simulink model "sfcndemo_dtype_io"  (Simulink 6.0)
settings: Solver=FixedStepDiscrete  StartTime=0.0  StopTime=10.0  RelTol=1e-3
settings Model: Creator=The MathWorks Inc.  LastModifiedBy=batserve  ExtModeAutoUpdateStatusClock=off
settings OptimizationCC: BlockReduction=off  BooleanDataType=off
settings DebuggingCC: CheckExecutionContextPreStartOutputMsg=on  CheckExecutionContextRuntimeOutputMsg=on  SolverPrmCheckMsg=none
settings HardwareCC: TargetUnknown=on

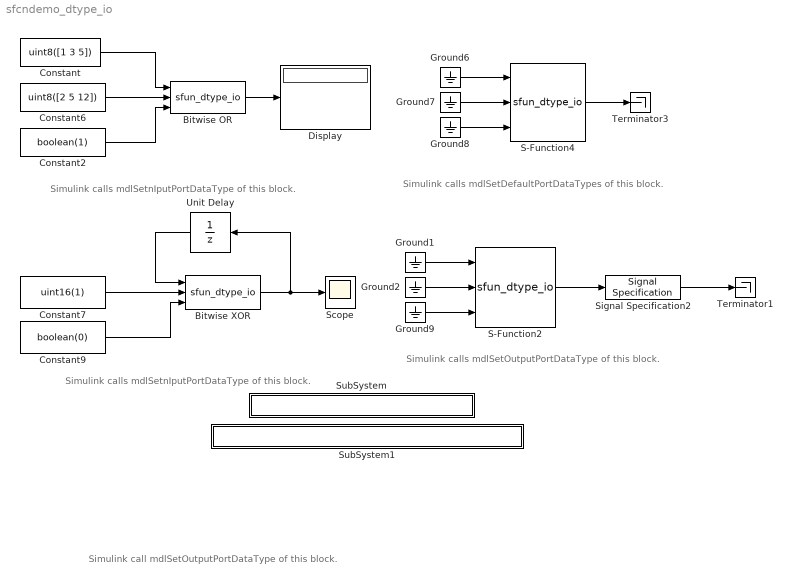
== system sfcndemo_dtype_io ==
  note: Simulink calls mdlSetDefaultPortDataTypes of this block.
  note: Simulink calls mdlSetOutputPortDataType of this block.
  note: Simulink call mdlSetOutputPortDataType of this block.
  note: Simulink calls mdlSetnIputPortDataType of this block.
  note: Simulink calls mdlSetnIputPortDataType of this block.
  Bitwise OR : S-Function  FunctionName=sfun_dtype_io
  Bitwise XOR : S-Function  FunctionName=sfun_dtype_io
  Constant : Constant  Value=uint8([1 3 5])
  Constant2 : Constant  Value=boolean(1)
  Constant6 : Constant  Value=uint8([2 5 12])
  Constant7 : Constant  Value=uint16(1)
  Constant9 : Constant  Value=boolean(0)
  Display : Display
  Ground{1..2,6..9} (6 alike) : Ground
  S-Function2 : S-Function  FunctionName=sfun_dtype_io
  S-Function4 : S-Function  FunctionName=sfun_dtype_io
  Scope : Scope
  Signal Specification2 : SignalSpecification  DataType=uint32
  SubSystem : Subsystem  PropExecContextAcrossSSBoundary=on
      settings: OpenFcn=edit(fullfile(matlabroot,'simulink','src','sfun_dtype_io.c'))
      mask Display: disp('matlabroot\simulink\src\sfun_dtype_io.c');
  SubSystem1 : Subsystem  PropExecContextAcrossSSBoundary=on
      settings: OpenFcn=edit(fullfile(matlabroot,'toolbox','simulink','blocks','tlc_c','sfun_dtype_io.tlc'))
      mask Display: disp('matlabroot\toolbox\simulink\blocks\tlc_c\sfun_dtype_io.tlc');
  Terminator1 : Terminator
  Terminator3 : Terminator
  Unit Delay : UnitDelay  Orientation=left
  wires:
  Constant/1 -> Bitwise OR/1
  Bitwise OR/1 -> Display/1
  Constant2/1 -> Bitwise OR/3
  Constant6/1 -> Bitwise OR/2
  Bitwise XOR/1 -> Unit Delay/1, Scope/1
  Constant9/1 -> Bitwise XOR/3
  Constant7/1 -> Bitwise XOR/2
  Unit Delay/1 -> Bitwise XOR/1
  Ground6/1 -> S-Function4/1
  S-Function4/1 -> Terminator3/1
  Ground7/1 -> S-Function4/2
  Ground8/1 -> S-Function4/3
  Ground1/1 -> S-Function2/1
  S-Function2/1 -> Signal Specification2/1
  Ground2/1 -> S-Function2/2
  Ground9/1 -> S-Function2/3
  Signal Specification2/1 -> Terminator1/1

== system sfcndemo_dtype_io/SubSystem ==

== system sfcndemo_dtype_io/SubSystem1 ==
